simulink model "Exam2"  (R2019b)
settings: Solver=FixedStepAuto  StartTime=0.0  StopTime=10.0  FixedStep=0.0001  RelTol=1e-3
values from neighbouring files (symbols this model uses):
  Kd = 1/(exp(T0/Kda)-1)    [exam.m]
  Kda = T1    (= 0.02)    [exam.m]
  Kp = Kpa    (= 33.3333333333)    [exam.m]
  Kpa = 1/(3*Tu)    (= 33.3333333333)    [exam.m]
  T0 = 0.01    [exam.m]
  T1 = 2*T0    (= 0.02)    [exam.m]
  Tur = T0/2    (= 0.005)    [exam.m]
settings Model: Creator=bedla  LastModifiedBy=bedla

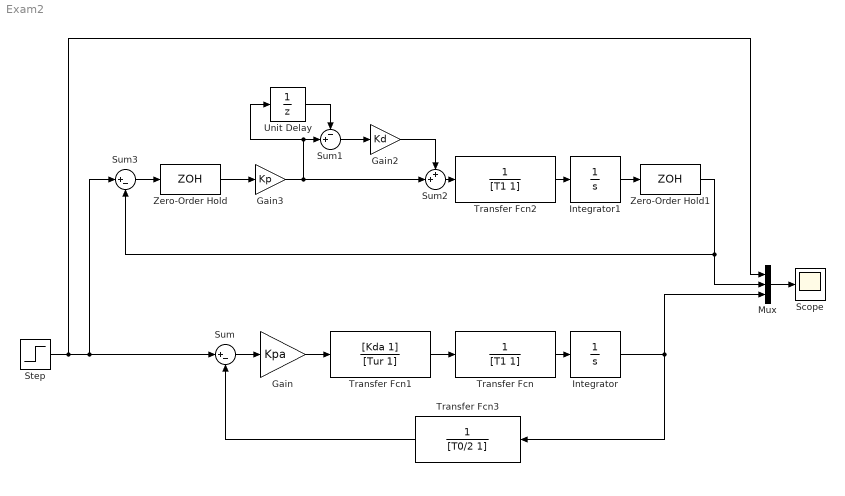
== system Exam2 ==
  Gain : Gain  Gain=Kpa
  Gain2 : Gain  Gain=Kd
  Gain3 : Gain  Gain=Kp
  Integrator : Integrator
  Integrator1 : Integrator
  Mux : Mux  Inputs=3
  Scope : Scope
  Step : Step  SampleTime=0
  Sum : Sum  Inputs=|+-
  Sum1 : Sum  Inputs=-+|
  Sum2 : Sum  Inputs=++|
  Sum3 : Sum  Inputs=|+-
  Transfer Fcn : TransferFcn  Denominator=[T1 1]
  Transfer Fcn1 : TransferFcn  Numerator=[Kda 1]  Denominator=[Tur 1]
  Transfer Fcn2 : TransferFcn  Denominator=[T1 1]
  Transfer Fcn3 : TransferFcn  Denominator=[T0/2 1]
  Unit Delay : UnitDelay  SampleTime=T0  HasFrameUpgradeWarning=on
  Zero-Order Hold : ZeroOrderHold  SampleTime=T0
  Zero-Order Hold1 : ZeroOrderHold  SampleTime=T0
  wires:
  Transfer Fcn/1 -> Integrator/1
  Transfer Fcn1/1 -> Transfer Fcn/1
  Gain/1 -> Transfer Fcn1/1
  Integrator/1 -> Mux/3, Transfer Fcn3/1
  Step/1 -> Mux/1, Sum3/1, Sum/1
  Sum/1 -> Gain/1
  Sum2/1 -> Transfer Fcn2/1
  Unit Delay/1 -> Sum1/1
  Gain2/1 -> Sum2/1
  Zero-Order Hold/1 -> Gain3/1
  Sum1/1 -> Gain2/1
  Sum3/1 -> Zero-Order Hold/1
  Zero-Order Hold1/1 -> Mux/2, Sum3/2
  Mux/1 -> Scope/1
  Gain3/1 -> Sum2/2, Unit Delay/1, Sum1/2
  Transfer Fcn2/1 -> Integrator1/1
  Integrator1/1 -> Zero-Order Hold1/1
  Transfer Fcn3/1 -> Sum/2
